simulink model "tank_linear_model"  (R2019b)
settings: Solver=VariableStepAuto  StartTime=0.0  StopTime=10.0  RelTol=1e-3
InitFcn:
  | load('workspace.mat')
values from neighbouring files (symbols this model uses):
  A = [-k1/(2*xe(1)^(1/2)), 0 ... (first row only)    [linearization.m]    (also in workspace.mat = [-0.0391932075235  0; 0.0391932075235  -0.0381972328031])
  b = [gamma1/(2*(beta1 + gamma1*ue(1))^(1/2)); 0]    [linearization.m]    (also in workspace.mat = [0.936765947069 0])
  h02 = 10.53    [equibrium.m]    (also in parameters.mat; workspace.mat)
  Ts = 0.5    [workspace.mat]
  ue = [ue1; ue2]    [equibrium.m]    (also in equibrium.mat = [1.87816229294 0]; workspace.mat = [1.87816229294 0])
  xe = [xe1; xe2]    [equibrium.m]    (also in equibrium.mat = [24.8812336392 25.53]; workspace.mat = [24.8812336392 25.53])
settings Model: Creator=tongk  LastModifiedBy=tongk

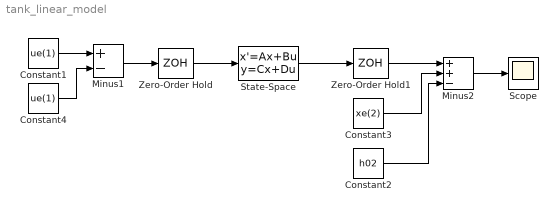
== system tank_linear_model ==
  Constant1 : Constant  Value=ue(1)
  Constant2 : Constant  Value=h02
  Constant3 : Constant  Value=xe(2)
  Constant4 : Constant  Value=ue(1)
  Minus1 : Sum  Inputs=+-
  Minus2 : Sum  Inputs=++-
  Scope : Scope
  State-Space : StateSpace  A=A  B=b  C=[0, 1]  D=0  InitialCondition=0
  Zero-Order Hold : ZeroOrderHold  SampleTime=Ts
  Zero-Order Hold1 : ZeroOrderHold  SampleTime=Ts
  wires:
  Zero-Order Hold/1 -> State-Space/1
  State-Space/1 -> Zero-Order Hold1/1
  Zero-Order Hold1/1 -> Minus2/1
  Constant3/1 -> Minus2/2
  Constant2/1 -> Minus2/3
  Minus2/1 -> Scope/1
  Constant1/1 -> Minus1/1
  Minus1/1 -> Zero-Order Hold/1
  Constant4/1 -> Minus1/2
